simulink model "LMS_FILTER_16_TAP"  (R2016a)
settings: Solver=VariableStepAuto  StartTime=0.0  StopTime=4000  RelTol=1e-3
libraries: dspsrcs4 x2, dspstat3 x2, dspmathops x1
settings Model: Creator=HP  LastModifiedBy=HP

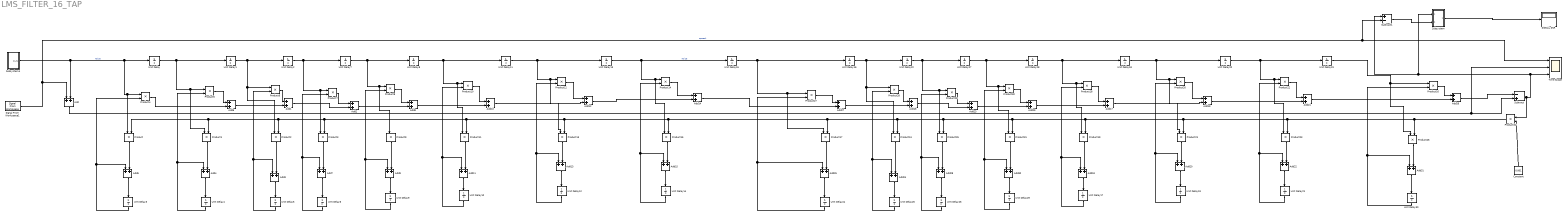
== system LMS_FILTER_16_TAP ==
  Add{,1..31} (32 alike) : Sum
  Constant : Constant  Value=0.001
  Product{,1..32} (33 alike) : Product
  "SIGNAL SNR " : Display
  Signal From Workspace1 : dspsrcs4/Signal From Workspace  X=m1  Ts=1  nsamps=1  OutputAfterFinalValue=Setting to zero  ignoreOrWarnInputAndFrameLengths=off  OutputFrames=off
  Subsystem : Subsystem
  Subsystem4 : Subsystem
  Subtract : Sum  Inputs=-+
  Subtract1 : Sum  Inputs=+-
  Time Scope : Scope  NumInputPorts=3
  Unit Delay{,1..30} (31 alike) : UnitDelay  SampleTime=-1
  wires:
  Unit Delay/1 -> Unit Delay1/1, Product1/1, Product5/1
  Unit Delay1/1 -> Product2/1, Product6/1, Unit Delay2/1
  Unit Delay2/1 -> Unit Delay7/1, Product7/1, Product3/1
  Unit Delay3/1 -> Add5/1, Product4/2
  Product/1 -> Add5/2
  Unit Delay4/1 -> Add4/1, Product5/2
  Add5/1 -> Unit Delay3/1
  Add4/1 -> Unit Delay4/1
  Product1/1 -> Add4/2
  Product5/1 -> Add6/1
  Product4/1 -> Add6/2
  Product2/1 -> Add3/2
  Unit Delay5/1 -> Add3/1, Product6/2
  Add3/1 -> Unit Delay5/1
  Product6/1 -> Add1/1
  Add6/1 -> Add1/2
  Unit Delay6/1 -> Add7/1, Product7/2
  Product3/1 -> Add7/2
  Product7/1 -> Add2/1
  Add1/1 -> Add2/2
  Add7/1 -> Unit Delay6/1
  Subsystem4/1(Out1) -> Add/2, Unit Delay/1, Product4/1, Product/1  "Noise"
  Unit Delay7/1 -> Unit Delay8/1, Product8/1, Product9/1
  Add9/1 -> Unit Delay9/1
  Unit Delay9/1 -> Add9/1, Product8/2
  Product8/1 -> Add8/1
  Add2/1 -> Add8/2
  Product9/1 -> Add9/2
  Unit Delay8/1 -> Unit Delay11/1, Product10/1, Product11/1
  Add11/1 -> Unit Delay10/1
  Unit Delay10/1 -> Add11/1, Product10/2
  Product10/1 -> Add10/1
  Add8/1 -> Add10/2
  Product11/1 -> Add11/2
  Unit Delay11/1 -> Unit Delay13/1, Product12/1, Product13/1
  Add13/1 -> Unit Delay12/1
  Unit Delay12/1 -> Add13/1, Product12/2
  Product12/1 -> Add12/1
  Add10/1 -> Add12/2
  Product13/1 -> Add13/2
  Add15/1 -> Unit Delay14/1
  Unit Delay14/1 -> Add15/1, Product14/2
  Product14/1 -> Add14/1
  Add12/1 -> Add14/2
  Product15/1 -> Add15/2
  Unit Delay15/1 -> Unit Delay16/1, Product27/1, Product17/1
  Unit Delay16/1 -> Product24/1, Product28/1, Unit Delay22/1
  Unit Delay22/1 -> Unit Delay27/1, Product29/1, Product25/1
  Unit Delay24/1 -> Add25/1, Product27/2
  Add25/1 -> Unit Delay24/1
  Product17/1 -> Add25/2
  Product27/1 -> Add27/1
  Product24/1 -> Add24/2
  Unit Delay25/1 -> Add24/1, Product28/2
  Add24/1 -> Unit Delay25/1
  Product28/1 -> Add16/1
  Add27/1 -> Add16/2
  Unit Delay26/1 -> Add28/1, Product29/2
  Product25/1 -> Add28/2
  Product29/1 -> Add23/1
  Add16/1 -> Add23/2
  Add28/1 -> Unit Delay26/1
  Unit Delay13/1 -> Unit Delay15/1, Product14/1, Product15/1  "Noise"
  Unit Delay27/1 -> Unit Delay28/1, Product30/1, Product31/1
  Add30/1 -> Unit Delay29/1
  Unit Delay29/1 -> Add30/1, Product30/2
  Product30/1 -> Add29/1
  Add23/1 -> Add29/2
  Product31/1 -> Add30/2
  Unit Delay28/1 -> Unit Delay18/1, Product18/1, Product19/1
  Add18/1 -> Unit Delay17/1
  Unit Delay17/1 -> Add18/1, Product18/2
  Product18/1 -> Add17/1
  Add29/1 -> Add17/2
  Product19/1 -> Add18/2
  Unit Delay18/1 -> Unit Delay20/1, Product20/1, Product21/1
  Add20/1 -> Unit Delay19/1
  Unit Delay19/1 -> Add20/1, Product20/2
  Product20/1 -> Add19/1
  Add17/1 -> Add19/2
  Product21/1 -> Add20/2
  Add22/1 -> Unit Delay21/1
  Unit Delay21/1 -> Add22/1, Product22/2
  Product22/1 -> Add21/1
  Add19/1 -> Add21/2
  Product23/1 -> Add22/2
  Add14/1 -> Add27/2
  Unit Delay20/1 -> Product22/1, Product23/1, Unit Delay23/1
  Unit Delay23/1 -> Product16/1, Product26/1
  Add31/1 -> Unit Delay30/1
  Unit Delay30/1 -> Add31/1, Product16/2
  Product16/1 -> Add26/1
  Add21/1 -> Add26/2
  Product26/1 -> Add31/2
  Add26/1 -> Subtract/1
  Add/1 -> Subtract/2, Time Scope/2
  Constant/1 -> Product32/2
  Product32/1 -> Product26/2, Product23/2, Product19/2, Product31/2, Product25/2, Product24/2, Product17/2, Product15/2, Product13/2, Product11/2, Product3/2, Product2/2, Product1/2, Product/2, Product21/2
  Signal From Workspace1/1 -> Add/1, Time Scope/1, Subtract1/2  "speech"
  Subtract/1 -> Product32/1, Time Scope/3, Subsystem/1(In1), Subtract1/1
  Subtract1/1 -> Subsystem/2(In2)
  Subsystem/1(Out1) -> "SIGNAL SNR "/1

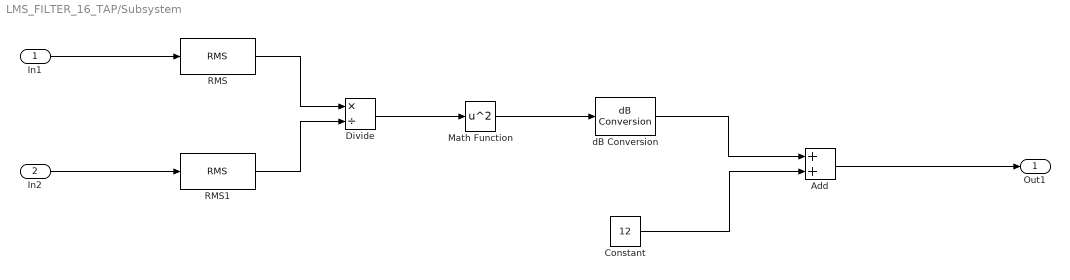
== system LMS_FILTER_16_TAP/Subsystem ==
  In1 : Inport
  In2 : Inport  Port=2
  Add : Sum
  Constant : Constant  Value=12
  Divide : Product  Inputs=*/
  Math Function : Math  Operator=square  OutputSignalType=real  SaturateOnIntegerOverflow=on
  RMS : dspstat3/RMS  run=on  reset_popup=None  InputProcessing=Columns as channels (frame based)  directionMode=Each column  dimension=1
  RMS1 : dspstat3/RMS  run=on  reset_popup=None  InputProcessing=Columns as channels (frame based)  directionMode=Each column  dimension=1
  dB Conversion : dspmathops/dB Conversion  dBtype=dB  intype=Amplitude  R=1  fuzz=off
  Out1 : Outport
  wires:
  RMS1/1 -> Divide/2
  dB Conversion/1 -> Add/1
  In1/1 -> RMS/1
  Divide/1 -> Math Function/1
  RMS/1 -> Divide/1
  In2/1 -> RMS1/1
  Add/1 -> Out1/1
  Constant/1 -> Add/2
  Math Function/1 -> dB Conversion/1

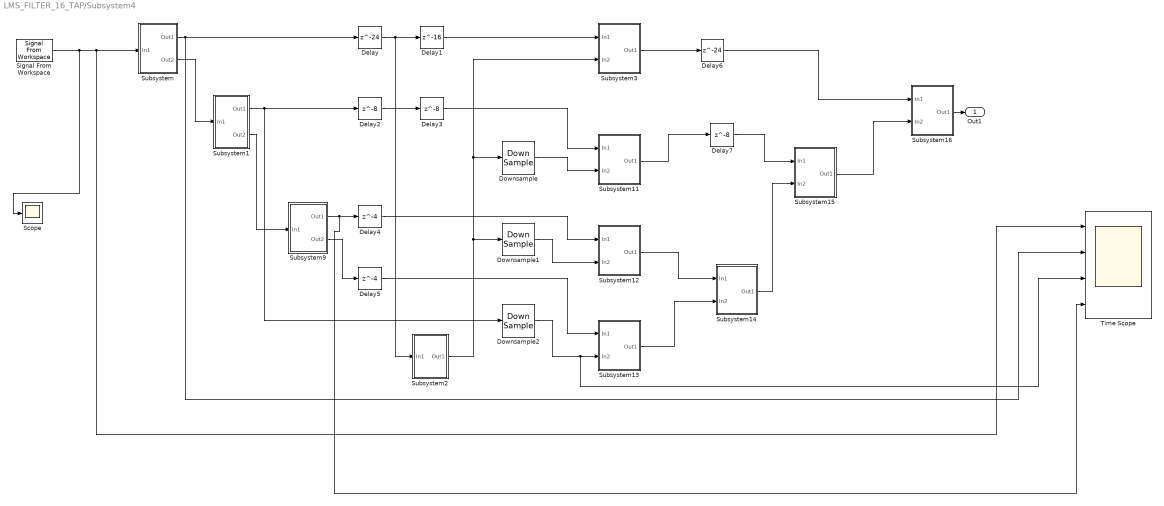
== system LMS_FILTER_16_TAP/Subsystem4 ==
  Delay : Delay  DelayLength=24  InitialCondition=0
  Delay1 : Delay  DelayLength=16  InitialCondition=0
  Delay2 : Delay  DelayLength=8  InitialCondition=0
  Delay3 : Delay  DelayLength=8  InitialCondition=0
  Delay4 : Delay  DelayLength=4  InitialCondition=0
  Delay5 : Delay  DelayLength=4  InitialCondition=0
  Delay6 : Delay  DelayLength=24  InitialCondition=0
  Delay7 : Delay  DelayLength=8  InitialCondition=0
  Downsample : DownSample  RateOptions=Allow multirate processing  ic=-1
  Downsample1 : DownSample  N=4  RateOptions=Allow multirate processing  ic=-1
  Downsample2 : DownSample  N=8  phase=1  ic=-1
  Scope : Scope
  Signal From Workspace : dspsrcs4/Signal From Workspace  X=y  Ts=1  nsamps=1  OutputAfterFinalValue=Setting to zero  ignoreOrWarnInputAndFrameLengths=off  OutputFrames=off
  Subsystem : Subsystem
  Subsystem1 : Subsystem
  Subsystem11 : Subsystem
  Subsystem12 : Subsystem
  Subsystem13 : Subsystem
  Subsystem14 : Subsystem
  Subsystem15 : Subsystem
  Subsystem16 : Subsystem
  Subsystem2 : Subsystem
  Subsystem3 : Subsystem
  Subsystem9 : Subsystem
  Time Scope : Scope  NumInputPorts=4
  Out1 : Outport
  wires:
  Subsystem1/2(Out2) -> Subsystem9/1(In1)
  Delay3/1 -> Subsystem11/1(In1)
  Downsample/1 -> Subsystem11/2(In2)
  Subsystem9/1(Out1) -> Time Scope/4, Delay4/1
  Subsystem/1(Out1) -> Delay/1, Time Scope/2
  Signal From Workspace/1 -> Scope/1, Time Scope/1, Subsystem/1(In1)
  Subsystem/2(Out2) -> Subsystem1/1(In1)
  Delay2/1 -> Delay3/1
  Subsystem11/1(Out1) -> Delay7/1
  Delay1/1 -> Subsystem3/1(In1)
  Delay/1 -> Subsystem2/1(In1), Delay1/1
  Delay4/1 -> Subsystem12/1(In1)
  Downsample2/1 -> Time Scope/3, Subsystem13/2(In2)
  Subsystem13/1(Out1) -> Subsystem14/2(In2)
  Subsystem3/1(Out1) -> Delay6/1
  Delay6/1 -> Subsystem16/1(In1)
  Subsystem1/1(Out1) -> Delay2/1, Downsample2/1
  Subsystem15/1(Out1) -> Subsystem16/2(In2)
  Subsystem14/1(Out1) -> Subsystem15/2(In2)
  Subsystem9/2(Out2) -> Delay5/1
  Downsample1/1 -> Subsystem12/2(In2)
  Delay5/1 -> Subsystem13/1(In1)
  Subsystem12/1(Out1) -> Subsystem14/1(In1)
  Delay7/1 -> Subsystem15/1(In1)
  Subsystem2/1(Out1) -> Downsample1/1, Subsystem3/2(In2), Downsample/1
  Subsystem16/1(Out1) -> Out1/1

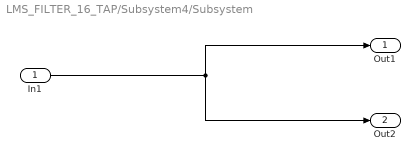
== system LMS_FILTER_16_TAP/Subsystem4/Subsystem ==
  In1 : Inport
  Out1 : Outport
  Out2 : Outport  Port=2
  wires:
  In1/1 -> Out1/1, Out2/1

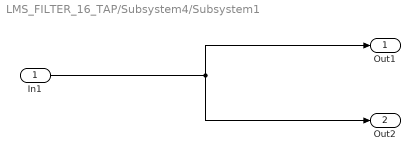
== system LMS_FILTER_16_TAP/Subsystem4/Subsystem1 ==
  In1 : Inport
  Out1 : Outport
  Out2 : Outport  Port=2
  wires:
  In1/1 -> Out1/1, Out2/1

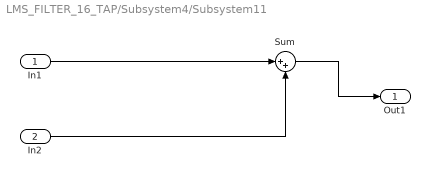
== system LMS_FILTER_16_TAP/Subsystem4/Subsystem11 ==
  In1 : Inport
  In2 : Inport  Port=2
  Sum : Sum  Inputs=|++
  Out1 : Outport
  wires:
  In1/1 -> Sum/1
  In2/1 -> Sum/2
  Sum/1 -> Out1/1

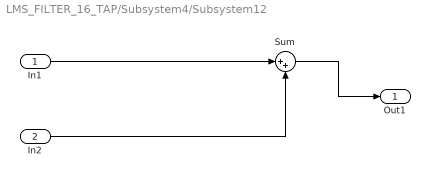
== system LMS_FILTER_16_TAP/Subsystem4/Subsystem12 ==
  In1 : Inport
  In2 : Inport  Port=2
  Sum : Sum  Inputs=|++
  Out1 : Outport
  wires:
  In1/1 -> Sum/1
  In2/1 -> Sum/2
  Sum/1 -> Out1/1

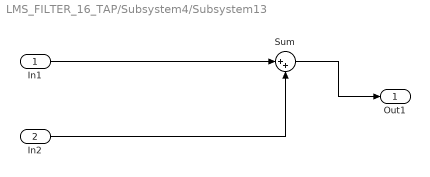
== system LMS_FILTER_16_TAP/Subsystem4/Subsystem13 ==
  In1 : Inport
  In2 : Inport  Port=2
  Sum : Sum  Inputs=|++
  Out1 : Outport
  wires:
  In1/1 -> Sum/1
  In2/1 -> Sum/2
  Sum/1 -> Out1/1

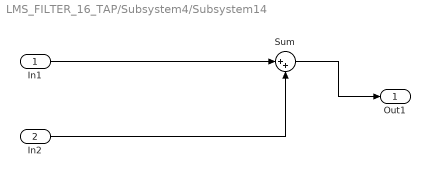
== system LMS_FILTER_16_TAP/Subsystem4/Subsystem14 ==
  In1 : Inport
  In2 : Inport  Port=2
  Sum : Sum  Inputs=|++
  Out1 : Outport
  wires:
  In1/1 -> Sum/1
  In2/1 -> Sum/2
  Sum/1 -> Out1/1

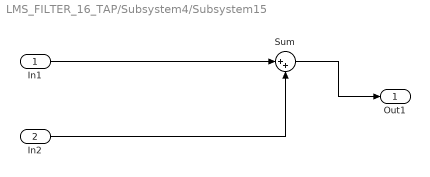
== system LMS_FILTER_16_TAP/Subsystem4/Subsystem15 ==
  In1 : Inport
  In2 : Inport  Port=2
  Sum : Sum  Inputs=|++
  Out1 : Outport
  wires:
  In1/1 -> Sum/1
  In2/1 -> Sum/2
  Sum/1 -> Out1/1

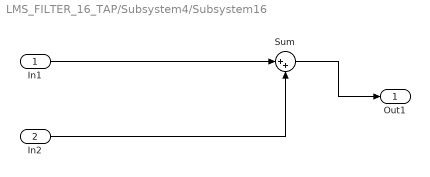
== system LMS_FILTER_16_TAP/Subsystem4/Subsystem16 ==
  In1 : Inport
  In2 : Inport  Port=2
  Sum : Sum  Inputs=|++
  Out1 : Outport
  wires:
  In1/1 -> Sum/1
  In2/1 -> Sum/2
  Sum/1 -> Out1/1

== system LMS_FILTER_16_TAP/Subsystem4/Subsystem2 ==
  In1 : Inport
  Out1 : Outport
  wires:
  In1/1 -> Out1/1

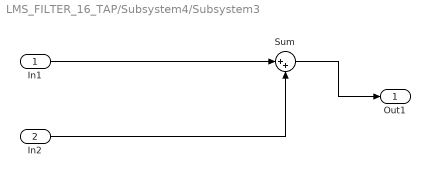
== system LMS_FILTER_16_TAP/Subsystem4/Subsystem3 ==
  In1 : Inport
  In2 : Inport  Port=2
  Sum : Sum  Inputs=|++
  Out1 : Outport
  wires:
  In1/1 -> Sum/1
  In2/1 -> Sum/2
  Sum/1 -> Out1/1

== system LMS_FILTER_16_TAP/Subsystem4/Subsystem9 ==
  In1 : Inport
  Out1 : Outport
  Out2 : Outport  Port=2
  wires:
  In1/1 -> Out1/1, Out2/1
